simulink model "Lab_4_Lab_5"  (R2016a)
settings: Solver=VariableStepAuto  SolverMode=SingleTasking  StartTime=0.0  StopTime=100  RelTol=1e-3
libraries: simulink x6, powerlib_extras x3
settings Model: Creator=WIN  LastModifiedBy=WIN
settings DebuggingCC: SFUnexpectedBacktrackingDiag=error  SFNoUnconditionalDefaultTransitionDiag=error
settings GRTTargetCC: TargetLangStandard=C99 (ISO)  GeneratePreprocessorConditionals=Use local settings
settings ConfigComp: CovMetricSettings=dwe  CovHtmlReporting=off  CovSaveCumulativeToWorkspaceVar=off  CovSaveSingleToWorkspaceVar=off  CovExternalEMLEnable=on

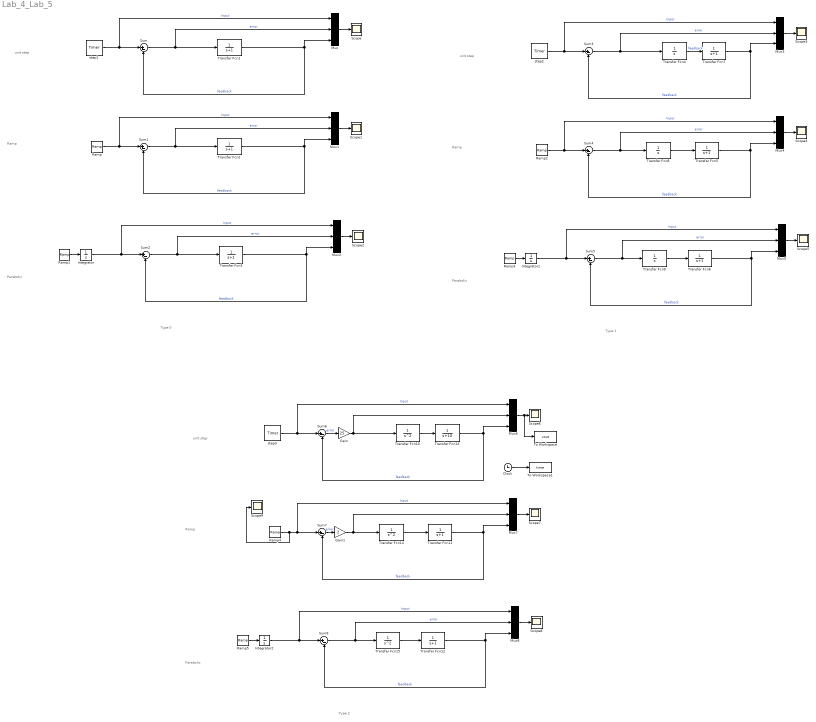
== system Lab_4_Lab_5 ==
  note: unit step
  note: Ramp
  note: Parabolic
  note: Type 0
  note: unit step
  note: Ramp
  note: Parabolic
  note: Type 1
  note: unit step
  note: Ramp
  note: Parabolic
  note: Type 2
  Clock : Clock
  Gain : Gain  Gain=25
  Gain1 : Gain  Gain=2
  Integrator : Integrator
  Integrator1 : Integrator
  Integrator2 : Integrator
  Mux{,1..8} (9 alike) : Mux  Inputs=3
  Ramp{,1..5} (6 alike) : simulink/Sources/Ramp  slope=1  start=0  X0=0
  Scope{,1..9} (10 alike) : Scope
  Sum{,1..8} (9 alike) : Sum  Inputs=|+-
  To Workspace : ToWorkspace  VariableName=vout  SampleTime=-1
  To Workspace1 : ToWorkspace  VariableName=time  SampleTime=-1
  Transfer Fcn{1..3,5..7,11..12} (8 alike) : TransferFcn  Denominator=[1 1]
  Transfer Fcn10 : TransferFcn  Denominator=[1 0 0]
  Transfer Fcn13 : TransferFcn  Denominator=[1 10]
  Transfer Fcn14 : TransferFcn  Denominator=[1 0 0]
  Transfer Fcn15 : TransferFcn  Denominator=[1 0 0]
  Transfer Fcn4 : TransferFcn  Denominator=[1 0]
  Transfer Fcn8 : TransferFcn  Denominator=[1 0]
  Transfer Fcn9 : TransferFcn  Denominator=[1 0]
  step1 : powerlib_extras/Control  Blocks/Timer  t=[0]  e=[1]
  step2 : powerlib_extras/Control  Blocks/Timer  t=[0]  e=[1]
  step3 : powerlib_extras/Control  Blocks/Timer  t=[0]  e=[1]
  wires:
  Sum/1 -> Mux/2, Transfer Fcn1/1  "error"
  Transfer Fcn1/1 -> Mux/3, Sum/2  "feedback"
  step1/1 -> Mux/1, Sum/1  "Input"
  Mux/1 -> Scope/1
  Mux1/1 -> Scope1/1
  Ramp/1 -> Sum1/1, Mux1/1  "Input"
  Transfer Fcn2/1 -> Sum1/2, Mux1/3  "feedback"
  Sum1/1 -> Transfer Fcn2/1, Mux1/2  "error"
  Sum2/1 -> Mux2/2, Transfer Fcn3/1  "error"
  Transfer Fcn3/1 -> Mux2/3, Sum2/2  "feedback"
  Integrator/1 -> Mux2/1, Sum2/1  "Input"
  Mux2/1 -> Scope2/1
  Ramp1/1 -> Integrator/1
  Ramp3/1 -> Integrator1/1
  Mux5/1 -> Scope5/1
  Integrator1/1 -> Sum5/1, Mux5/1  "Input"
  Transfer Fcn6/1 -> Sum5/2, Mux5/3  "feedback"
  Sum5/1 -> Transfer Fcn9/1, Mux5/2  "error"
  Sum4/1 -> Mux4/2, Transfer Fcn8/1  "error"
  Transfer Fcn5/1 -> Mux4/3, Sum4/2  "feedback"
  Ramp2/1 -> Mux4/1, Sum4/1  "Input"
  Mux4/1 -> Scope4/1
  Mux3/1 -> Scope3/1
  step2/1 -> Sum3/1, Mux3/1  "Input"
  Transfer Fcn4/1 -> Transfer Fcn7/1  "feedback"
  Sum3/1 -> Transfer Fcn4/1, Mux3/2  "error"
  Transfer Fcn7/1 -> Sum3/2, Mux3/3  "feedback"
  Transfer Fcn8/1 -> Transfer Fcn5/1
  Transfer Fcn9/1 -> Transfer Fcn6/1
  Transfer Fcn15/1 -> Transfer Fcn12/1
  Transfer Fcn14/1 -> Transfer Fcn11/1
  Transfer Fcn13/1 -> Mux6/3, Sum6/2  "feedback"
  Sum6/1 -> Gain/1  "error"
  Transfer Fcn10/1 -> Transfer Fcn13/1
  step3/1 -> Mux6/1, Sum6/1  "Input"
  Mux6/1 -> To Workspace/1, Scope6/1
  Mux7/1 -> Scope7/1
  Ramp4/1 -> Scope9/1, Sum7/1, Mux7/1  "Input"
  Transfer Fcn11/1 -> Sum7/2, Mux7/3  "feedback"
  Sum7/1 -> Gain1/1  "error"
  Sum8/1 -> Transfer Fcn15/1, Mux8/2  "error"
  Transfer Fcn12/1 -> Mux8/3, Sum8/2  "feedback"
  Integrator2/1 -> Mux8/1, Sum8/1  "Input"
  Mux8/1 -> Scope8/1
  Ramp5/1 -> Integrator2/1
  Gain/1 -> Transfer Fcn10/1, Mux6/2
  Gain1/1 -> Transfer Fcn14/1, Mux7/2
  Clock/1 -> To Workspace1/1
